simulink model "PanelSolarSeguidor_comp"  (R2022b)
settings: Solver=VariableStepAuto  StartTime=0.0  StopTime=10.0  RelTol=1e-3
model workspace (MAT data in the model file):
  amplitude_sinewave = 10000
  bias_sinewave = 0
  const = 10000
  final_step = 10000
  frec_sinewave = 1
  intial_step = 0
  phase_sinewave = 0
  selector = 1
  steptime_step = 1
values from neighbouring files (symbols this model uses):
  beta = 0.785398163397    [PanelSolarSeguidor.mat]    (also in PanelSolarSeguidor_3D.m)
  d = [0 1 0]    [PanelSolarSeguidor.mat]    (also in PanelSolarSeguidor_3D.m = Ry * [d(1);d(2);d(3)])
  initial_pendiente = 0    [PanelSolarSeguidor.mat]    (also in PanelSolarSeguidor_3D.m)
  Kd = 5    [PanelSolarSeguidor.mat]    (also in PanelSolarSeguidor_3D.m)
  Kf = 1.835    [PanelSolarSeguidor.mat]    (also in PanelSolarSeguidor_3D.m)
  Kg = 20    [PanelSolarSeguidor.mat]    (also in PanelSolarSeguidor_3D.m)
  Kt = 1.835    [PanelSolarSeguidor.mat]    (also in PanelSolarSeguidor_3D.m)
  l = 2.18    [PanelSolarSeguidor.mat]    (also in PanelSolarSeguidor_3D.m)
  L = 0.1042    [PanelSolarSeguidor.mat]    (also in PanelSolarSeguidor_3D.m)
  m = 24.5    [PanelSolarSeguidor.mat]    (also in PanelSolarSeguidor_3D.m)
  pendiente_rampa = 10000    [PanelSolarSeguidor.mat]    (also in PanelSolarSeguidor_3D.m)
  R = 3.05    [PanelSolarSeguidor.mat]    (also in PanelSolarSeguidor_3D.m)
  sampletime_sinewave = 0    [PanelSolarSeguidor.mat]    (also in PanelSolarSeguidor_3D.m)
  sampletime_step = 0    [PanelSolarSeguidor.mat]    (also in PanelSolarSeguidor_3D.m)
  w = 0.996    [PanelSolarSeguidor.mat]    (also in PanelSolarSeguidor_3D.m)
libraries: simulink x2
settings Model: Creator=marte  LastModifiedBy=anton

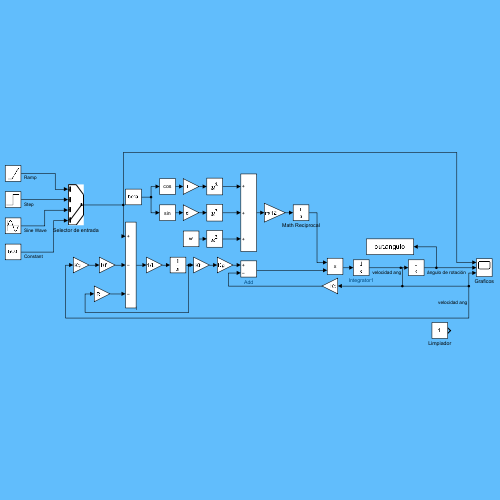
[thumbnail: Simulink's stored preview of the top-level diagram]
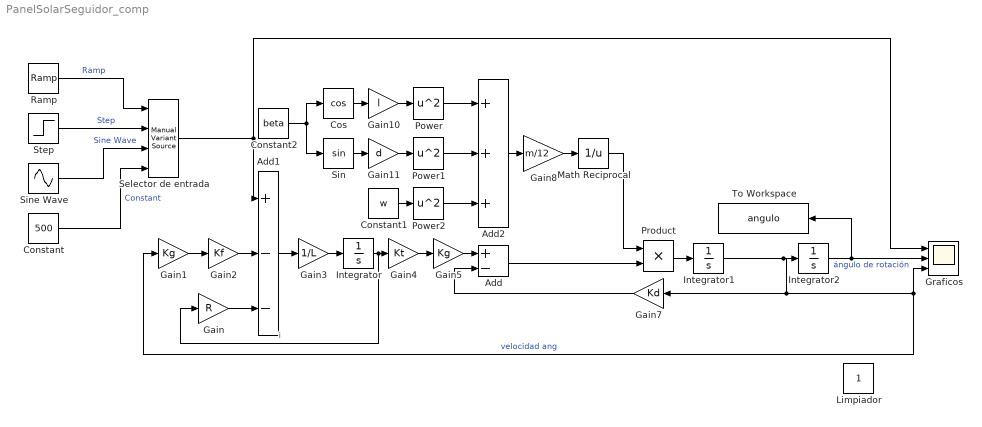
== system PanelSolarSeguidor_comp ==
  Add : Sum  Inputs=+-
  Add1 : Sum  Inputs=+--
  Add2 : Sum  Inputs=+++
  Constant : Constant  Value=500
  Constant1 : Constant  Value=w
  Constant2 : Constant  Value=beta
  Cos : Trigonometry  Operator=cos
  Gain : Gain  Gain=R
  Gain1 : Gain  Gain=Kg
  Gain10 : Gain  Gain=l
  Gain11 : Gain  Gain=d
  Gain2 : Gain  Gain=Kf
  Gain3 : Gain  Gain=1/L
  Gain4 : Gain  Gain=Kt
  Gain5 : Gain  Gain=Kg
  Gain7 : Gain  Gain=Kd
  Gain8 : Gain  Gain=m/12
  Graficos : Scope  NumInputPorts=3
  Integrator : Integrator
  Integrator1 : Integrator
  Integrator2 : Integrator
  Limpiador : Constant
  Math Reciprocal : Math  Operator=reciprocal  SignedPower=on
  Power : Math  Operator=square
  Power1 : Math  Operator=square
  Power2 : Math  Operator=square
  Product : Product
  Ramp : simulink/Sources/Ramp  slope=pendiente_rampa  start=start_time_pendiente  InitialOutput=initial_pendiente
  Selector de entrada : simulink/Signal Routing/Manual Variant Source  NumChoices=4  LabelModeActiveChoice=V_4
  Sin : Trigonometry
  Sine Wave : Sin  Amplitude=amplitude_sinewave  Bias=bias_sinewave  Frequency=frec_sinewave  Phase=phase_sinewave  SampleTime=sampletime_sinewave
  Step : Step  Time=steptime_step  Before=intial_step  After=final_step  SampleTime=sampletime_step
  To Workspace : ToWorkspace  VariableName=angulo  SaveFormat=Timeseries  SampleTime=-1
  wires:
  Gain2/1 -> Add1/2
  Integrator/1 -> Gain4/1, Gain/1  "i"
  Gain5/1 -> Add/1
  Gain1/1 -> Gain2/1
  Integrator2/1 -> Graficos/2, To Workspace/1  "ángulo de rotación"
  Gain/1 -> Add1/3
  Add1/1 -> Gain3/1
  Integrator1/1 -> Gain1/1, Graficos/3, Gain7/1, Integrator2/1  "velocidad ang"
  Gain4/1 -> Gain5/1
  Gain3/1 -> Integrator/1
  Gain7/1 -> Add/2
  Power/1 -> Add2/1
  Power1/1 -> Add2/2
  Power2/1 -> Add2/3
  Gain8/1 -> Math Reciprocal/1
  Add2/1 -> Gain8/1
  Constant1/1 -> Power2/1
  Constant2/1 -> Sin/1, Cos/1
  Cos/1 -> Gain10/1
  Sin/1 -> Gain11/1
  Gain10/1 -> Power/1
  Gain11/1 -> Power1/1
  Add/1 -> Product/2
  Math Reciprocal/1 -> Product/1
  Product/1 -> Integrator1/1
  Selector de entrada/1 -> Graficos/1, Add1/1
  Ramp/1 -> Selector de entrada/1  "Ramp"
  Step/1 -> Selector de entrada/2  "Step"
  Sine Wave/1 -> Selector de entrada/3  "Sine Wave"
  Constant/1 -> Selector de entrada/4  "Constant"
